simulink model "P_I_PI_Controller"  (R2023a)
settings: Solver=VariableStepAuto  StartTime=0.0  StopTime=100  MaxStep=0.001  RelTol=1e-3
settings Model: Creator=Mohamed Ezzelrgal  LastModifiedBy=Mohamed Ezzelrgal

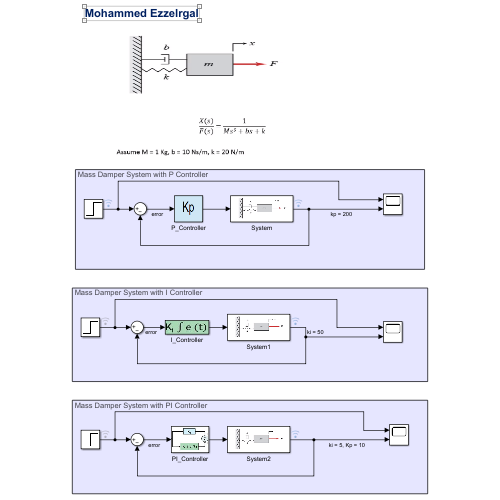
[thumbnail: Simulink's stored preview of the top-level diagram]
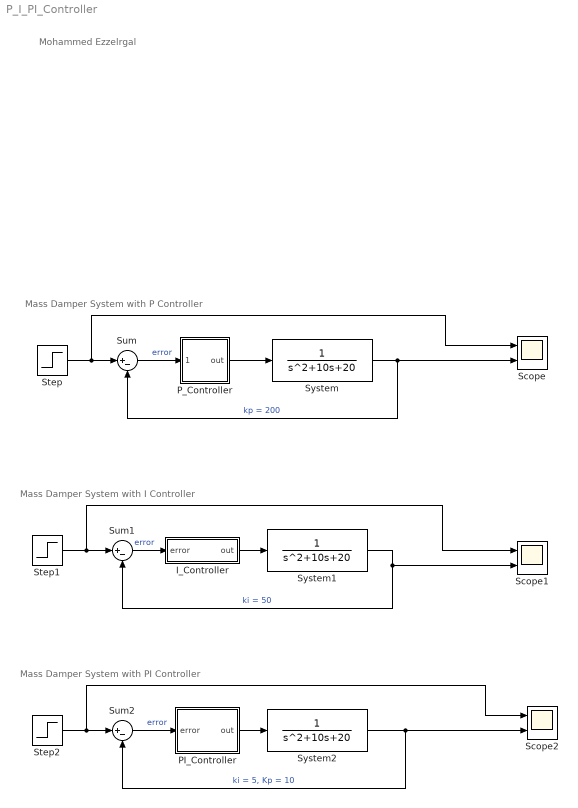
== system P_I_PI_Controller ==
  note: Mohammed Ezzelrgal
  note: Mass Damper System with P Controller
  note: Mass Damper System with I Controller
  note: Mass Damper System with PI Controller
  I_Controller : Subsystem
      mask Display: image('C:\Users\User\Desktop\i.png'); % Use "Edit Image" on toolstrip to change.
  PI_Controller : Subsystem
      mask Display: image('C:\Users\User\Desktop\pi.png'); % Use "Edit Image" on toolstrip to change.
  P_Controller : Subsystem
      mask Display: image('C:\Users\User\Desktop\p.png'); % Use "Edit Image" on toolstrip to change.
  Scope : Scope  NumInputPorts=2
  Scope1 : Scope  NumInputPorts=2
  Scope2 : Scope  NumInputPorts=2
  Step : Step  SampleTime=0
  Step1 : Step  SampleTime=0
  Step2 : Step  SampleTime=0
  Sum : Sum  Inputs=|+-
  Sum1 : Sum  Inputs=|+-
  Sum2 : Sum  Inputs=|+-
  System : TransferFcn  Denominator=[1 10 20]
      mask Display: image('ffff.png');
  System1 : TransferFcn  Denominator=[1 10 20]
      mask Display: image('ffff.png');
  System2 : TransferFcn  Denominator=[1 10 20]
      mask Display: image('ffff.png');
  wires:
  P_Controller/1(out) -> System/1
  Step/1 -> Scope/1, Sum/1
  Sum/1 -> P_Controller/1(error)  "error"
  System/1 -> Sum/2, Scope/2  "kp = 200"
  System1/1 -> Scope1/2, Sum1/2  "ki = 50"
  Sum1/1 -> I_Controller/1(error)  "error"
  Step1/1 -> Sum1/1, Scope1/1
  I_Controller/1(out) -> System1/1
  PI_Controller/1(out) -> System2/1
  Step2/1 -> Scope2/1, Sum2/1
  Sum2/1 -> PI_Controller/1(error)  "error"
  System2/1 -> Sum2/2, Scope2/2  "ki = 5, Kp = 10"

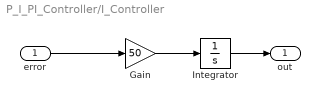
== system P_I_PI_Controller/I_Controller ==
  error : Inport
  Gain : Gain  Gain=50
  Integrator : Integrator
  out : Outport
  wires:
  Gain/1 -> Integrator/1
  error/1 -> Gain/1
  Integrator/1 -> out/1

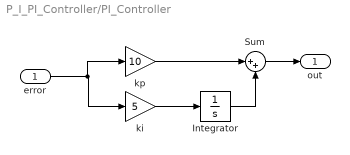
== system P_I_PI_Controller/PI_Controller ==
  error : Inport
  Integrator : Integrator
  Sum : Sum  Inputs=|++
  ki : Gain  Gain=5
  kp : Gain  Gain=10
  out : Outport
  wires:
  error/1 -> kp/1, ki/1
  ki/1 -> Integrator/1
  Sum/1 -> out/1
  Integrator/1 -> Sum/2
  kp/1 -> Sum/1

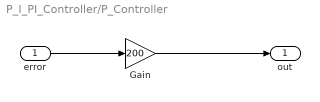
== system P_I_PI_Controller/P_Controller ==
  error : Inport
  Gain : Gain  Gain=200
  out : Outport
  wires:
  error/1 -> Gain/1
  Gain/1 -> out/1
